simulink model "p4_system_arch_master"  (R2020a)
settings: Solver=VariableStepAuto  StartTime=0.0  StopTime=10.0  RelTol=1e-3
(part 8 of 11)

== system p4_system_arch_master/System 8 : Suspension and Vibration Damping System /motor mount system/support system/Bracket ==

== system p4_system_arch_master/System 8 : Suspension and Vibration Damping System /motor mount system/support system/elastomer ==

== system p4_system_arch_master/System 1 : Electric Motor System /Stator System /1.3 AC HV Connection System  /1.3.1 Connection System /Phase U Connection Ring ==

== system p4_system_arch_master/System 1 : Electric Motor System /Stator System /1.3 AC HV Connection System  /1.3.1 Connection System /Phase V Connection Ring ==

== system p4_system_arch_master/System 1 : Electric Motor System /Stator System /1.3 AC HV Connection System  /1.3.1 Connection System /Phase W Connection Ring ==

== system p4_system_arch_master/System 1 : Electric Motor System /Stator System /1.3 AC HV Connection System  /Isolation System/Isolator Rotor Phase U ==

== system p4_system_arch_master/System 1 : Electric Motor System /Stator System /1.3 AC HV Connection System  /Isolation System/Isolator Rotor Phase U to Phase V ==

== system p4_system_arch_master/System 1 : Electric Motor System /Stator System /1.3 AC HV Connection System  /Isolation System/Isolator Rotor Phase V to Phase W ==

== system p4_system_arch_master/System 10 : Electrical Distribution System /10.1 HV Distribution System /10.1.1	HV DC vehicle interface system/10.1.1.1	HV DC to vehicle connection system/10.1.1.1.1	HV DC Male Connector ==

== system p4_system_arch_master/System 10 : Electrical Distribution System /10.1 HV Distribution System /10.1.1	HV DC vehicle interface system/10.1.1.2	HV DC to inverter connection system/10.1.1.2.1	HV DC Cable Lug "+" ==

== system p4_system_arch_master/System 10 : Electrical Distribution System /10.1 HV Distribution System /10.1.1	HV DC vehicle interface system/10.1.1.2	HV DC to inverter connection system/10.1.1.2.2	HV DC Cable Lug "-"  ==

== system p4_system_arch_master/System 10 : Electrical Distribution System /10.1 HV Distribution System /10.1.1	HV DC vehicle interface system/10.1.1.2	HV DC to inverter connection system/10.1.1.2.3	HV DC Cable Lug "+" Screw ==

== system p4_system_arch_master/System 10 : Electrical Distribution System /10.1 HV Distribution System /10.1.1	HV DC vehicle interface system/10.1.1.2	HV DC to inverter connection system/10.1.1.2.4	HV DC Cable Lug "-" Screw ==

== system p4_system_arch_master/System 10 : Electrical Distribution System /10.1 HV Distribution System /10.1.1	HV DC vehicle interface system/10.1.1.2	HV DC to inverter connection system/10.1.1.2.5	HV DC Cable Lug "+" Washer ==

== system p4_system_arch_master/System 10 : Electrical Distribution System /10.1 HV Distribution System /10.1.1	HV DC vehicle interface system/10.1.1.2	HV DC to inverter connection system/10.1.1.2.6	HV DC Cable Lug "-" Washer ==

== system p4_system_arch_master/System 10 : Electrical Distribution System /10.1 HV Distribution System /10.1.1	HV DC vehicle interface system/10.1.1.3	HV DC Wiring system/10.1.1.3.1	HV DC Wire "+" ==

== system p4_system_arch_master/System 10 : Electrical Distribution System /10.1 HV Distribution System /10.1.1	HV DC vehicle interface system/10.1.1.3	HV DC Wiring system/10.1.1.3.2	HV DC Wire "+" Shielding Braid ==

== system p4_system_arch_master/System 10 : Electrical Distribution System /10.1 HV Distribution System /10.1.1	HV DC vehicle interface system/10.1.1.3	HV DC Wiring system/10.1.1.3.3	HV DC Wire "+" Insulation ==

== system p4_system_arch_master/System 10 : Electrical Distribution System /10.1 HV Distribution System /10.1.1	HV DC vehicle interface system/10.1.1.3	HV DC Wiring system/10.1.1.3.4	HV DC Wire "-" ==

== system p4_system_arch_master/System 10 : Electrical Distribution System /10.1 HV Distribution System /10.1.1	HV DC vehicle interface system/10.1.1.3	HV DC Wiring system/10.1.1.3.5	HV DC Wire "-" Shielding Braid ==

== system p4_system_arch_master/System 10 : Electrical Distribution System /10.1 HV Distribution System /10.1.1	HV DC vehicle interface system/10.1.1.3	HV DC Wiring system/10.1.1.3.6	HV DC Wire "-" Insulation ==

== system p4_system_arch_master/System 10 : Electrical Distribution System /10.1 HV Distribution System /10.1.2	HV AC 3-Phase System (Busbars)/10.1.2.1	HV AC U Busbar System/10.1.2.1.1	HV AC U busbar ==

== system p4_system_arch_master/System 10 : Electrical Distribution System /10.1 HV Distribution System /10.1.2	HV AC 3-Phase System (Busbars)/10.1.2.1	HV AC U Busbar System/10.1.2.1.2	HV AC U busbar to motor bolt ==

== system p4_system_arch_master/System 10 : Electrical Distribution System /10.1 HV Distribution System /10.1.2	HV AC 3-Phase System (Busbars)/10.1.2.1	HV AC U Busbar System/10.1.2.1.3	HV AC U busbar to inverter bolt ==

== system p4_system_arch_master/System 10 : Electrical Distribution System /10.1 HV Distribution System /10.1.2	HV AC 3-Phase System (Busbars)/10.1.2.1	HV AC U Busbar System/10.1.2.1.4	HV AC U busbar to motor washer ==

== system p4_system_arch_master/System 10 : Electrical Distribution System /10.1 HV Distribution System /10.1.2	HV AC 3-Phase System (Busbars)/10.1.2.1	HV AC U Busbar System/10.1.2.1.5	HV AC U busbar to inverter washer ==

== system p4_system_arch_master/System 10 : Electrical Distribution System /10.1 HV Distribution System /10.1.2	HV AC 3-Phase System (Busbars)/10.1.2.1	HV AC U Busbar System/10.1.2.1.6	HV AC U busbar Insulation ==

== system p4_system_arch_master/System 10 : Electrical Distribution System /10.1 HV Distribution System /10.1.2	HV AC 3-Phase System (Busbars)/10.1.2.2	HV AC V Busbar System/10.1.2.2.2	HV AC V busbar to motor bolt ==

== system p4_system_arch_master/System 10 : Electrical Distribution System /10.1 HV Distribution System /10.1.2	HV AC 3-Phase System (Busbars)/10.1.2.2	HV AC V Busbar System/10.1.2.2.3	HV AC V busbar to inverter bolt ==

== system p4_system_arch_master/System 10 : Electrical Distribution System /10.1 HV Distribution System /10.1.2	HV AC 3-Phase System (Busbars)/10.1.2.2	HV AC V Busbar System/10.1.2.2.4	HV AC V busbar to motor washer ==

== system p4_system_arch_master/System 10 : Electrical Distribution System /10.1 HV Distribution System /10.1.2	HV AC 3-Phase System (Busbars)/10.1.2.2	HV AC V Busbar System/10.1.2.2.5	HV AC V busbar to inverter washer ==

== system p4_system_arch_master/System 10 : Electrical Distribution System /10.1 HV Distribution System /10.1.2	HV AC 3-Phase System (Busbars)/10.1.2.2	HV AC V Busbar System/10.1.2.2.6	HV AC V busbar Insulation ==

== system p4_system_arch_master/System 10 : Electrical Distribution System /10.1 HV Distribution System /10.1.2	HV AC 3-Phase System (Busbars)/10.1.2.3	HV AC W Busbar System/10.1.2.3.1	HV AC W busbar ==

== system p4_system_arch_master/System 10 : Electrical Distribution System /10.1 HV Distribution System /10.1.2	HV AC 3-Phase System (Busbars)/10.1.2.3	HV AC W Busbar System/10.1.2.3.2	HV AC W busbar to motor bolt ==

== system p4_system_arch_master/System 10 : Electrical Distribution System /10.1 HV Distribution System /10.1.2	HV AC 3-Phase System (Busbars)/10.1.2.3	HV AC W Busbar System/10.1.2.3.3	HV AC W busbar to inverter bolt ==

== system p4_system_arch_master/System 10 : Electrical Distribution System /10.1 HV Distribution System /10.1.2	HV AC 3-Phase System (Busbars)/10.1.2.3	HV AC W Busbar System/10.1.2.3.4	HV AC W busbar to motor washer ==

== system p4_system_arch_master/System 10 : Electrical Distribution System /10.1 HV Distribution System /10.1.2	HV AC 3-Phase System (Busbars)/10.1.2.3	HV AC W Busbar System/10.1.2.3.5	HV AC W busbar to inverter washer ==

== system p4_system_arch_master/System 10 : Electrical Distribution System /10.1 HV Distribution System /10.1.2	HV AC 3-Phase System (Busbars)/10.1.2.3	HV AC W Busbar System/10.1.2.3.6	HV AC W busbar Insulation ==

== system p4_system_arch_master/System 10 : Electrical Distribution System /10.2 LV Distribution System /10.2.1	Internal LV Loom System/10.2.1.1	Inverter to Motor LV loom system/10.2.1.1.01	Motor LV loom to inverter PCB connector ==

== system p4_system_arch_master/System 10 : Electrical Distribution System /10.2 LV Distribution System /10.2.1	Internal LV Loom System/10.2.1.1	Inverter to Motor LV loom system/PT100 #1 Wire System ==
  "10.2.1.1.18\tPT100 #1 Wire \"Ex+\"" : Subsystem
      settings: PortSchema="{\"entries\":[{\"content\":{\"headerSize\":26,\"margin\":15,\"minimumSpacing\":25,\"sides\":[{\"content\":{\"connectorIds\":[]},\"type\":\"ConnectorPlacement.EquallySpacedRectSide\",\"uuid\":\"f8ee33a9-954f-44c6-a821-b5353f3278fa\"},{\"content\":{\"connectorIds\":[],\"side\":\"RIGHT\"},\"type\":\"ConnectorPlacement.EquallySpacedRectSide\",\"uuid\":\"385f1e4f-1c89-4afc-9c19-76a078cf90bc\"},{\"content\":{\"connectorIds\":[],\"side\":\"TOP\"},\"type\":\"ConnectorPlacement.EquallySpacedRectSide\",\"uuid\":\"fc91fa49-46f5-4ba7-960e-7bda5e0416d1\"}]},\"type\":\"ConnectorPlacement.EquallySpacedConnector\",\"uuid\":\"4bf08bc6-c7ce-47fb-af04-cd9d2b5f8092\"}],\"packageUris\":[\"http://schema.mathworks.com/mf0/Connector/19700101\"],\"version\":\"1.0\"}"
  "10.2.1.1.19\tPT100 #1 Wire \"Ex-\"" : Subsystem
      settings: PortSchema="{\"entries\":[{\"content\":{\"headerSize\":26,\"margin\":15,\"minimumSpacing\":25,\"sides\":[{\"content\":{\"connectorIds\":[]},\"type\":\"ConnectorPlacement.EquallySpacedRectSide\",\"uuid\":\"f8ee33a9-954f-44c6-a821-b5353f3278fa\"},{\"content\":{\"connectorIds\":[],\"side\":\"RIGHT\"},\"type\":\"ConnectorPlacement.EquallySpacedRectSide\",\"uuid\":\"385f1e4f-1c89-4afc-9c19-76a078cf90bc\"},{\"content\":{\"connectorIds\":[],\"side\":\"TOP\"},\"type\":\"ConnectorPlacement.EquallySpacedRectSide\",\"uuid\":\"fc91fa49-46f5-4ba7-960e-7bda5e0416d1\"}]},\"type\":\"ConnectorPlacement.EquallySpacedConnector\",\"uuid\":\"4bf08bc6-c7ce-47fb-af04-cd9d2b5f8092\"}],\"packageUris\":[\"http://schema.mathworks.com/mf0/Connector/19700101\"],\"version\":\"1.0\"}"
  "10.2.1.1.20\tPT100 #1 Wire \"Ex+\" Insulation" : Subsystem
      settings: PortSchema="{\"entries\":[{\"content\":{\"headerSize\":26,\"margin\":15,\"minimumSpacing\":25,\"sides\":[{\"content\":{\"connectorIds\":[]},\"type\":\"ConnectorPlacement.EquallySpacedRectSide\",\"uuid\":\"f8ee33a9-954f-44c6-a821-b5353f3278fa\"},{\"content\":{\"connectorIds\":[],\"side\":\"RIGHT\"},\"type\":\"ConnectorPlacement.EquallySpacedRectSide\",\"uuid\":\"385f1e4f-1c89-4afc-9c19-76a078cf90bc\"},{\"content\":{\"connectorIds\":[],\"side\":\"TOP\"},\"type\":\"ConnectorPlacement.EquallySpacedRectSide\",\"uuid\":\"fc91fa49-46f5-4ba7-960e-7bda5e0416d1\"}]},\"type\":\"ConnectorPlacement.EquallySpacedConnector\",\"uuid\":\"4bf08bc6-c7ce-47fb-af04-cd9d2b5f8092\"}],\"packageUris\":[\"http://schema.mathworks.com/mf0/Connector/19700101\"],\"version\":\"1.0\"}"
  "10.2.1.1.21\tPT100 #1 Wire \"Ex-\" Insulation" : Subsystem
      settings: PortSchema="{\"entries\":[{\"content\":{\"headerSize\":26,\"margin\":15,\"minimumSpacing\":25,\"sides\":[{\"content\":{\"connectorIds\":[]},\"type\":\"ConnectorPlacement.EquallySpacedRectSide\",\"uuid\":\"f8ee33a9-954f-44c6-a821-b5353f3278fa\"},{\"content\":{\"connectorIds\":[],\"side\":\"RIGHT\"},\"type\":\"ConnectorPlacement.EquallySpacedRectSide\",\"uuid\":\"385f1e4f-1c89-4afc-9c19-76a078cf90bc\"},{\"content\":{\"connectorIds\":[],\"side\":\"TOP\"},\"type\":\"ConnectorPlacement.EquallySpacedRectSide\",\"uuid\":\"fc91fa49-46f5-4ba7-960e-7bda5e0416d1\"}]},\"type\":\"ConnectorPlacement.EquallySpacedConnector\",\"uuid\":\"4bf08bc6-c7ce-47fb-af04-cd9d2b5f8092\"}],\"packageUris\":[\"http://schema.mathworks.com/mf0/Connector/19700101\"],\"version\":\"1.0\"}"
  "10.2.1.1.22\tPT100 #1 Wire pair \"Ex\" shielding braid" : Subsystem
      settings: PortSchema="{\"entries\":[{\"content\":{\"headerSize\":26,\"margin\":15,\"minimumSpacing\":25,\"sides\":[{\"content\":{\"connectorIds\":[]},\"type\":\"ConnectorPlacement.EquallySpacedRectSide\",\"uuid\":\"f8ee33a9-954f-44c6-a821-b5353f3278fa\"},{\"content\":{\"connectorIds\":[],\"side\":\"RIGHT\"},\"type\":\"ConnectorPlacement.EquallySpacedRectSide\",\"uuid\":\"385f1e4f-1c89-4afc-9c19-76a078cf90bc\"},{\"content\":{\"connectorIds\":[],\"side\":\"TOP\"},\"type\":\"ConnectorPlacement.EquallySpacedRectSide\",\"uuid\":\"fc91fa49-46f5-4ba7-960e-7bda5e0416d1\"}]},\"type\":\"ConnectorPlacement.EquallySpacedConnector\",\"uuid\":\"4bf08bc6-c7ce-47fb-af04-cd9d2b5f8092\"}],\"packageUris\":[\"http://schema.mathworks.com/mf0/Connector/19700101\"],\"version\":\"1.0\"}"

== system p4_system_arch_master/System 10 : Electrical Distribution System /10.2 LV Distribution System /10.2.1	Internal LV Loom System/10.2.1.1	Inverter to Motor LV loom system/PT100 #2 Wire System ==
  "10.2.1.1.23\tPT100 #2 Wire \"Ex+\"" : Subsystem
      settings: PortSchema="{\"entries\":[{\"content\":{\"headerSize\":26,\"margin\":15,\"minimumSpacing\":25,\"sides\":[{\"content\":{\"connectorIds\":[]},\"type\":\"ConnectorPlacement.EquallySpacedRectSide\",\"uuid\":\"f8ee33a9-954f-44c6-a821-b5353f3278fa\"},{\"content\":{\"connectorIds\":[],\"side\":\"RIGHT\"},\"type\":\"ConnectorPlacement.EquallySpacedRectSide\",\"uuid\":\"385f1e4f-1c89-4afc-9c19-76a078cf90bc\"},{\"content\":{\"connectorIds\":[],\"side\":\"TOP\"},\"type\":\"ConnectorPlacement.EquallySpacedRectSide\",\"uuid\":\"fc91fa49-46f5-4ba7-960e-7bda5e0416d1\"}]},\"type\":\"ConnectorPlacement.EquallySpacedConnector\",\"uuid\":\"4bf08bc6-c7ce-47fb-af04-cd9d2b5f8092\"}],\"packageUris\":[\"http://schema.mathworks.com/mf0/Connector/19700101\"],\"version\":\"1.0\"}"
  "10.2.1.1.24\tPT100 #2 Wire \"Ex-\"" : Subsystem
      settings: PortSchema="{\"entries\":[{\"content\":{\"headerSize\":26,\"margin\":15,\"minimumSpacing\":25,\"sides\":[{\"content\":{\"connectorIds\":[]},\"type\":\"ConnectorPlacement.EquallySpacedRectSide\",\"uuid\":\"f8ee33a9-954f-44c6-a821-b5353f3278fa\"},{\"content\":{\"connectorIds\":[],\"side\":\"RIGHT\"},\"type\":\"ConnectorPlacement.EquallySpacedRectSide\",\"uuid\":\"385f1e4f-1c89-4afc-9c19-76a078cf90bc\"},{\"content\":{\"connectorIds\":[],\"side\":\"TOP\"},\"type\":\"ConnectorPlacement.EquallySpacedRectSide\",\"uuid\":\"fc91fa49-46f5-4ba7-960e-7bda5e0416d1\"}]},\"type\":\"ConnectorPlacement.EquallySpacedConnector\",\"uuid\":\"4bf08bc6-c7ce-47fb-af04-cd9d2b5f8092\"}],\"packageUris\":[\"http://schema.mathworks.com/mf0/Connector/19700101\"],\"version\":\"1.0\"}"
  "10.2.1.1.25\tPT100 #2 Wire \"Ex+\" Insulation" : Subsystem
      settings: PortSchema="{\"entries\":[{\"content\":{\"headerSize\":26,\"margin\":15,\"minimumSpacing\":25,\"sides\":[{\"content\":{\"connectorIds\":[]},\"type\":\"ConnectorPlacement.EquallySpacedRectSide\",\"uuid\":\"f8ee33a9-954f-44c6-a821-b5353f3278fa\"},{\"content\":{\"connectorIds\":[],\"side\":\"RIGHT\"},\"type\":\"ConnectorPlacement.EquallySpacedRectSide\",\"uuid\":\"385f1e4f-1c89-4afc-9c19-76a078cf90bc\"},{\"content\":{\"connectorIds\":[],\"side\":\"TOP\"},\"type\":\"ConnectorPlacement.EquallySpacedRectSide\",\"uuid\":\"fc91fa49-46f5-4ba7-960e-7bda5e0416d1\"}]},\"type\":\"ConnectorPlacement.EquallySpacedConnector\",\"uuid\":\"4bf08bc6-c7ce-47fb-af04-cd9d2b5f8092\"}],\"packageUris\":[\"http://schema.mathworks.com/mf0/Connector/19700101\"],\"version\":\"1.0\"}"
  "10.2.1.1.26\tPT100 #2 Wire \"Ex-\" Insulation" : Subsystem
      settings: PortSchema="{\"entries\":[{\"content\":{\"headerSize\":26,\"margin\":15,\"minimumSpacing\":25,\"sides\":[{\"content\":{\"connectorIds\":[]},\"type\":\"ConnectorPlacement.EquallySpacedRectSide\",\"uuid\":\"f8ee33a9-954f-44c6-a821-b5353f3278fa\"},{\"content\":{\"connectorIds\":[],\"side\":\"RIGHT\"},\"type\":\"ConnectorPlacement.EquallySpacedRectSide\",\"uuid\":\"385f1e4f-1c89-4afc-9c19-76a078cf90bc\"},{\"content\":{\"connectorIds\":[],\"side\":\"TOP\"},\"type\":\"ConnectorPlacement.EquallySpacedRectSide\",\"uuid\":\"fc91fa49-46f5-4ba7-960e-7bda5e0416d1\"}]},\"type\":\"ConnectorPlacement.EquallySpacedConnector\",\"uuid\":\"4bf08bc6-c7ce-47fb-af04-cd9d2b5f8092\"}],\"packageUris\":[\"http://schema.mathworks.com/mf0/Connector/19700101\"],\"version\":\"1.0\"}"
  "10.2.1.1.27\tPT100 #2 Wire pair \"Ex\" shielding braid" : Subsystem
      settings: PortSchema="{\"entries\":[{\"content\":{\"headerSize\":26,\"margin\":15,\"minimumSpacing\":25,\"sides\":[{\"content\":{\"connectorIds\":[]},\"type\":\"ConnectorPlacement.EquallySpacedRectSide\",\"uuid\":\"f8ee33a9-954f-44c6-a821-b5353f3278fa\"},{\"content\":{\"connectorIds\":[],\"side\":\"RIGHT\"},\"type\":\"ConnectorPlacement.EquallySpacedRectSide\",\"uuid\":\"385f1e4f-1c89-4afc-9c19-76a078cf90bc\"},{\"content\":{\"connectorIds\":[],\"side\":\"TOP\"},\"type\":\"ConnectorPlacement.EquallySpacedRectSide\",\"uuid\":\"fc91fa49-46f5-4ba7-960e-7bda5e0416d1\"}]},\"type\":\"ConnectorPlacement.EquallySpacedConnector\",\"uuid\":\"4bf08bc6-c7ce-47fb-af04-cd9d2b5f8092\"}],\"packageUris\":[\"http://schema.mathworks.com/mf0/Connector/19700101\"],\"version\":\"1.0\"}"

== system p4_system_arch_master/System 10 : Electrical Distribution System /10.2 LV Distribution System /10.2.1	Internal LV Loom System/10.2.1.1	Inverter to Motor LV loom system/Resolver sensor System ==
  10.2.1.1.02	Resolver sensor connector : Subsystem
      settings: PortSchema="{\"entries\":[{\"content\":{\"headerSize\":26,\"margin\":15,\"minimumSpacing\":25,\"sides\":[{\"content\":{\"connectorIds\":[]},\"type\":\"ConnectorPlacement.EquallySpacedRectSide\",\"uuid\":\"f8ee33a9-954f-44c6-a821-b5353f3278fa\"},{\"content\":{\"connectorIds\":[],\"side\":\"RIGHT\"},\"type\":\"ConnectorPlacement.EquallySpacedRectSide\",\"uuid\":\"385f1e4f-1c89-4afc-9c19-76a078cf90bc\"},{\"content\":{\"connectorIds\":[],\"side\":\"TOP\"},\"type\":\"ConnectorPlacement.EquallySpacedRectSide\",\"uuid\":\"fc91fa49-46f5-4ba7-960e-7bda5e0416d1\"}]},\"type\":\"ConnectorPlacement.EquallySpacedConnector\",\"uuid\":\"4bf08bc6-c7ce-47fb-af04-cd9d2b5f8092\"}],\"packageUris\":[\"http://schema.mathworks.com/mf0/Connector/19700101\"],\"version\":\"1.0\"}"
  10.2.1.1.03	Resolver sensor  Wires : Subsystem
      settings: PortSchema="{\"entries\":[{\"content\":{\"headerSize\":26,\"margin\":15,\"minimumSpacing\":25,\"sides\":[{\"content\":{\"connectorIds\":[]},\"type\":\"ConnectorPlacement.EquallySpacedRectSide\",\"uuid\":\"f8ee33a9-954f-44c6-a821-b5353f3278fa\"},{\"content\":{\"connectorIds\":[],\"side\":\"RIGHT\"},\"type\":\"ConnectorPlacement.EquallySpacedRectSide\",\"uuid\":\"385f1e4f-1c89-4afc-9c19-76a078cf90bc\"},{\"content\":{\"connectorIds\":[],\"side\":\"TOP\"},\"type\":\"ConnectorPlacement.EquallySpacedRectSide\",\"uuid\":\"fc91fa49-46f5-4ba7-960e-7bda5e0416d1\"}]},\"type\":\"ConnectorPlacement.EquallySpacedConnector\",\"uuid\":\"4bf08bc6-c7ce-47fb-af04-cd9d2b5f8092\"}],\"packageUris\":[\"http://schema.mathworks.com/mf0/Connector/19700101\"],\"version\":\"1.0\"}"

== system p4_system_arch_master/System 10 : Electrical Distribution System /10.2 LV Distribution System /10.2.1	Internal LV Loom System/10.2.1.2	Inverter to Inverter LV connector loom system/10.2.1.2.01	Inverter LV external connector ==

== system p4_system_arch_master/System 10 : Electrical Distribution System /10.2 LV Distribution System /10.2.1	Internal LV Loom System/10.2.1.2	Inverter to Inverter LV connector loom system/10.2.1.2.02	Inverter internal loom to PCB connector ==

== system p4_system_arch_master/System 10 : Electrical Distribution System /10.2 LV Distribution System /10.2.1	Internal LV Loom System/10.2.1.2	Inverter to Inverter LV connector loom system/Inverter Internal Wires ==
  CAN1_H Wire : Subsystem
      settings: PortSchema="{\"entries\":[{\"content\":{\"headerSize\":26,\"margin\":15,\"minimumSpacing\":25,\"sides\":[{\"content\":{\"connectorIds\":[]},\"type\":\"ConnectorPlacement.EquallySpacedRectSide\",\"uuid\":\"f8ee33a9-954f-44c6-a821-b5353f3278fa\"},{\"content\":{\"connectorIds\":[],\"side\":\"RIGHT\"},\"type\":\"ConnectorPlacement.EquallySpacedRectSide\",\"uuid\":\"385f1e4f-1c89-4afc-9c19-76a078cf90bc\"},{\"content\":{\"connectorIds\":[],\"side\":\"TOP\"},\"type\":\"ConnectorPlacement.EquallySpacedRectSide\",\"uuid\":\"fc91fa49-46f5-4ba7-960e-7bda5e0416d1\"}]},\"type\":\"ConnectorPlacement.EquallySpacedConnector\",\"uuid\":\"4bf08bc6-c7ce-47fb-af04-cd9d2b5f8092\"}],\"packageUris\":[\"http://schema.mathworks.com/mf0/Connector/19700101\"],\"version\":\"1.0\"}"
  CAN1_L Wire : Subsystem
      settings: PortSchema="{\"entries\":[{\"content\":{\"headerSize\":26,\"margin\":15,\"minimumSpacing\":25,\"sides\":[{\"content\":{\"connectorIds\":[]},\"type\":\"ConnectorPlacement.EquallySpacedRectSide\",\"uuid\":\"f8ee33a9-954f-44c6-a821-b5353f3278fa\"},{\"content\":{\"connectorIds\":[],\"side\":\"RIGHT\"},\"type\":\"ConnectorPlacement.EquallySpacedRectSide\",\"uuid\":\"385f1e4f-1c89-4afc-9c19-76a078cf90bc\"},{\"content\":{\"connectorIds\":[],\"side\":\"TOP\"},\"type\":\"ConnectorPlacement.EquallySpacedRectSide\",\"uuid\":\"fc91fa49-46f5-4ba7-960e-7bda5e0416d1\"}]},\"type\":\"ConnectorPlacement.EquallySpacedConnector\",\"uuid\":\"4bf08bc6-c7ce-47fb-af04-cd9d2b5f8092\"}],\"packageUris\":[\"http://schema.mathworks.com/mf0/Connector/19700101\"],\"version\":\"1.0\"}"
  CAN2_H Wire : Subsystem
      settings: PortSchema="{\"entries\":[{\"content\":{\"headerSize\":26,\"margin\":15,\"minimumSpacing\":25,\"sides\":[{\"content\":{\"connectorIds\":[]},\"type\":\"ConnectorPlacement.EquallySpacedRectSide\",\"uuid\":\"f8ee33a9-954f-44c6-a821-b5353f3278fa\"},{\"content\":{\"connectorIds\":[],\"side\":\"RIGHT\"},\"type\":\"ConnectorPlacement.EquallySpacedRectSide\",\"uuid\":\"385f1e4f-1c89-4afc-9c19-76a078cf90bc\"},{\"content\":{\"connectorIds\":[],\"side\":\"TOP\"},\"type\":\"ConnectorPlacement.EquallySpacedRectSide\",\"uuid\":\"fc91fa49-46f5-4ba7-960e-7bda5e0416d1\"}]},\"type\":\"ConnectorPlacement.EquallySpacedConnector\",\"uuid\":\"4bf08bc6-c7ce-47fb-af04-cd9d2b5f8092\"}],\"packageUris\":[\"http://schema.mathworks.com/mf0/Connector/19700101\"],\"version\":\"1.0\"}"
  "CAN2_L Wire " : Subsystem
      settings: PortSchema="{\"entries\":[{\"content\":{\"headerSize\":26,\"margin\":15,\"minimumSpacing\":25,\"sides\":[{\"content\":{\"connectorIds\":[]},\"type\":\"ConnectorPlacement.EquallySpacedRectSide\",\"uuid\":\"f8ee33a9-954f-44c6-a821-b5353f3278fa\"},{\"content\":{\"connectorIds\":[],\"side\":\"RIGHT\"},\"type\":\"ConnectorPlacement.EquallySpacedRectSide\",\"uuid\":\"385f1e4f-1c89-4afc-9c19-76a078cf90bc\"},{\"content\":{\"connectorIds\":[],\"side\":\"TOP\"},\"type\":\"ConnectorPlacement.EquallySpacedRectSide\",\"uuid\":\"fc91fa49-46f5-4ba7-960e-7bda5e0416d1\"}]},\"type\":\"ConnectorPlacement.EquallySpacedConnector\",\"uuid\":\"4bf08bc6-c7ce-47fb-af04-cd9d2b5f8092\"}],\"packageUris\":[\"http://schema.mathworks.com/mf0/Connector/19700101\"],\"version\":\"1.0\"}"
  DIN1 Wire : Subsystem
      settings: PortSchema="{\"entries\":[{\"content\":{\"headerSize\":26,\"margin\":15,\"minimumSpacing\":25,\"sides\":[{\"content\":{\"connectorIds\":[]},\"type\":\"ConnectorPlacement.EquallySpacedRectSide\",\"uuid\":\"f8ee33a9-954f-44c6-a821-b5353f3278fa\"},{\"content\":{\"connectorIds\":[],\"side\":\"RIGHT\"},\"type\":\"ConnectorPlacement.EquallySpacedRectSide\",\"uuid\":\"385f1e4f-1c89-4afc-9c19-76a078cf90bc\"},{\"content\":{\"connectorIds\":[],\"side\":\"TOP\"},\"type\":\"ConnectorPlacement.EquallySpacedRectSide\",\"uuid\":\"fc91fa49-46f5-4ba7-960e-7bda5e0416d1\"}]},\"type\":\"ConnectorPlacement.EquallySpacedConnector\",\"uuid\":\"4bf08bc6-c7ce-47fb-af04-cd9d2b5f8092\"}],\"packageUris\":[\"http://schema.mathworks.com/mf0/Connector/19700101\"],\"version\":\"1.0\"}"
  DIN2 Wire : Subsystem
      settings: PortSchema="{\"entries\":[{\"content\":{\"headerSize\":26,\"margin\":15,\"minimumSpacing\":25,\"sides\":[{\"content\":{\"connectorIds\":[]},\"type\":\"ConnectorPlacement.EquallySpacedRectSide\",\"uuid\":\"f8ee33a9-954f-44c6-a821-b5353f3278fa\"},{\"content\":{\"connectorIds\":[],\"side\":\"RIGHT\"},\"type\":\"ConnectorPlacement.EquallySpacedRectSide\",\"uuid\":\"385f1e4f-1c89-4afc-9c19-76a078cf90bc\"},{\"content\":{\"connectorIds\":[],\"side\":\"TOP\"},\"type\":\"ConnectorPlacement.EquallySpacedRectSide\",\"uuid\":\"fc91fa49-46f5-4ba7-960e-7bda5e0416d1\"}]},\"type\":\"ConnectorPlacement.EquallySpacedConnector\",\"uuid\":\"4bf08bc6-c7ce-47fb-af04-cd9d2b5f8092\"}],\"packageUris\":[\"http://schema.mathworks.com/mf0/Connector/19700101\"],\"version\":\"1.0\"}"
  DOUT1 Wire : Subsystem
      settings: PortSchema="{\"entries\":[{\"content\":{\"headerSize\":26,\"margin\":15,\"minimumSpacing\":25,\"sides\":[{\"content\":{\"connectorIds\":[]},\"type\":\"ConnectorPlacement.EquallySpacedRectSide\",\"uuid\":\"f8ee33a9-954f-44c6-a821-b5353f3278fa\"},{\"content\":{\"connectorIds\":[],\"side\":\"RIGHT\"},\"type\":\"ConnectorPlacement.EquallySpacedRectSide\",\"uuid\":\"385f1e4f-1c89-4afc-9c19-76a078cf90bc\"},{\"content\":{\"connectorIds\":[],\"side\":\"TOP\"},\"type\":\"ConnectorPlacement.EquallySpacedRectSide\",\"uuid\":\"fc91fa49-46f5-4ba7-960e-7bda5e0416d1\"}]},\"type\":\"ConnectorPlacement.EquallySpacedConnector\",\"uuid\":\"4bf08bc6-c7ce-47fb-af04-cd9d2b5f8092\"}],\"packageUris\":[\"http://schema.mathworks.com/mf0/Connector/19700101\"],\"version\":\"1.0\"}"
  DOUT2 Wire : Subsystem
      settings: PortSchema="{\"entries\":[{\"content\":{\"headerSize\":26,\"margin\":15,\"minimumSpacing\":25,\"sides\":[{\"content\":{\"connectorIds\":[]},\"type\":\"ConnectorPlacement.EquallySpacedRectSide\",\"uuid\":\"f8ee33a9-954f-44c6-a821-b5353f3278fa\"},{\"content\":{\"connectorIds\":[],\"side\":\"RIGHT\"},\"type\":\"ConnectorPlacement.EquallySpacedRectSide\",\"uuid\":\"385f1e4f-1c89-4afc-9c19-76a078cf90bc\"},{\"content\":{\"connectorIds\":[],\"side\":\"TOP\"},\"type\":\"ConnectorPlacement.EquallySpacedRectSide\",\"uuid\":\"fc91fa49-46f5-4ba7-960e-7bda5e0416d1\"}]},\"type\":\"ConnectorPlacement.EquallySpacedConnector\",\"uuid\":\"4bf08bc6-c7ce-47fb-af04-cd9d2b5f8092\"}],\"packageUris\":[\"http://schema.mathworks.com/mf0/Connector/19700101\"],\"version\":\"1.0\"}"
  ETH_N Wire : Subsystem
      settings: PortSchema="{\"entries\":[{\"content\":{\"headerSize\":26,\"margin\":15,\"minimumSpacing\":25,\"sides\":[{\"content\":{\"connectorIds\":[]},\"type\":\"ConnectorPlacement.EquallySpacedRectSide\",\"uuid\":\"f8ee33a9-954f-44c6-a821-b5353f3278fa\"},{\"content\":{\"connectorIds\":[],\"side\":\"RIGHT\"},\"type\":\"ConnectorPlacement.EquallySpacedRectSide\",\"uuid\":\"385f1e4f-1c89-4afc-9c19-76a078cf90bc\"},{\"content\":{\"connectorIds\":[],\"side\":\"TOP\"},\"type\":\"ConnectorPlacement.EquallySpacedRectSide\",\"uuid\":\"fc91fa49-46f5-4ba7-960e-7bda5e0416d1\"}]},\"type\":\"ConnectorPlacement.EquallySpacedConnector\",\"uuid\":\"4bf08bc6-c7ce-47fb-af04-cd9d2b5f8092\"}],\"packageUris\":[\"http://schema.mathworks.com/mf0/Connector/19700101\"],\"version\":\"1.0\"}"
  ETH_P Wire : Subsystem
      settings: PortSchema="{\"entries\":[{\"content\":{\"headerSize\":26,\"margin\":15,\"minimumSpacing\":25,\"sides\":[{\"content\":{\"connectorIds\":[]},\"type\":\"ConnectorPlacement.EquallySpacedRectSide\",\"uuid\":\"f8ee33a9-954f-44c6-a821-b5353f3278fa\"},{\"content\":{\"connectorIds\":[],\"side\":\"RIGHT\"},\"type\":\"ConnectorPlacement.EquallySpacedRectSide\",\"uuid\":\"385f1e4f-1c89-4afc-9c19-76a078cf90bc\"},{\"content\":{\"connectorIds\":[],\"side\":\"TOP\"},\"type\":\"ConnectorPlacement.EquallySpacedRectSide\",\"uuid\":\"fc91fa49-46f5-4ba7-960e-7bda5e0416d1\"}]},\"type\":\"ConnectorPlacement.EquallySpacedConnector\",\"uuid\":\"4bf08bc6-c7ce-47fb-af04-cd9d2b5f8092\"}],\"packageUris\":[\"http://schema.mathworks.com/mf0/Connector/19700101\"],\"version\":\"1.0\"}"
  "GND Wire " : Subsystem
      settings: PortSchema="{\"entries\":[{\"content\":{\"headerSize\":26,\"margin\":15,\"minimumSpacing\":25,\"sides\":[{\"content\":{\"connectorIds\":[]},\"type\":\"ConnectorPlacement.EquallySpacedRectSide\",\"uuid\":\"f8ee33a9-954f-44c6-a821-b5353f3278fa\"},{\"content\":{\"connectorIds\":[],\"side\":\"RIGHT\"},\"type\":\"ConnectorPlacement.EquallySpacedRectSide\",\"uuid\":\"385f1e4f-1c89-4afc-9c19-76a078cf90bc\"},{\"content\":{\"connectorIds\":[],\"side\":\"TOP\"},\"type\":\"ConnectorPlacement.EquallySpacedRectSide\",\"uuid\":\"fc91fa49-46f5-4ba7-960e-7bda5e0416d1\"}]},\"type\":\"ConnectorPlacement.EquallySpacedConnector\",\"uuid\":\"4bf08bc6-c7ce-47fb-af04-cd9d2b5f8092\"}],\"packageUris\":[\"http://schema.mathworks.com/mf0/Connector/19700101\"],\"version\":\"1.0\"}"
  VCC Wire : Subsystem
      settings: PortSchema="{\"entries\":[{\"content\":{\"headerSize\":26,\"margin\":15,\"minimumSpacing\":25,\"sides\":[{\"content\":{\"connectorIds\":[]},\"type\":\"ConnectorPlacement.EquallySpacedRectSide\",\"uuid\":\"f8ee33a9-954f-44c6-a821-b5353f3278fa\"},{\"content\":{\"connectorIds\":[],\"side\":\"RIGHT\"},\"type\":\"ConnectorPlacement.EquallySpacedRectSide\",\"uuid\":\"385f1e4f-1c89-4afc-9c19-76a078cf90bc\"},{\"content\":{\"connectorIds\":[],\"side\":\"TOP\"},\"type\":\"ConnectorPlacement.EquallySpacedRectSide\",\"uuid\":\"fc91fa49-46f5-4ba7-960e-7bda5e0416d1\"}]},\"type\":\"ConnectorPlacement.EquallySpacedConnector\",\"uuid\":\"4bf08bc6-c7ce-47fb-af04-cd9d2b5f8092\"}],\"packageUris\":[\"http://schema.mathworks.com/mf0/Connector/19700101\"],\"version\":\"1.0\"}"

== system p4_system_arch_master/System 10 : Electrical Distribution System /10.2 LV Distribution System /10.2.1	Internal LV Loom System/10.2.1.3	Internal LV loom restraining system/10.2.1.3.1	Cable clips ==

== system p4_system_arch_master/System 10 : Electrical Distribution System /10.2 LV Distribution System /10.2.2	External LV Loom System/10.2.2.1	External LV loom connectors system/10.2.2.1.01	Main LV connector IDU to vehicle  ==

== system p4_system_arch_master/System 10 : Electrical Distribution System /10.2 LV Distribution System /10.2.2	External LV Loom System/10.2.2.1	External LV loom connectors system/10.2.2.1.02	Inverter cable connector ==

== system p4_system_arch_master/System 10 : Electrical Distribution System /10.2 LV Distribution System /10.2.2	External LV Loom System/10.2.2.1	External LV loom connectors system/10.2.2.1.03	I//O module X1 cable connector ==

== system p4_system_arch_master/System 10 : Electrical Distribution System /10.2 LV Distribution System /10.2.2	External LV Loom System/10.2.2.1	External LV loom connectors system/10.2.2.1.04	I//O module X2 cable connector ==

== system p4_system_arch_master/System 10 : Electrical Distribution System /10.2 LV Distribution System /10.2.2	External LV Loom System/10.2.2.1	External LV loom connectors system/10.2.2.1.05	Oil temperature sensor connector ==

== system p4_system_arch_master/System 10 : Electrical Distribution System /10.2 LV Distribution System /10.2.2	External LV Loom System/10.2.2.1	External LV loom connectors system/10.2.2.1.06	Input speed sensor connector ==

== system p4_system_arch_master/System 10 : Electrical Distribution System /10.2 LV Distribution System /10.2.2	External LV Loom System/10.2.2.1	External LV loom connectors system/10.2.2.1.07	Output speed sensor connector ==

== system p4_system_arch_master/System 10 : Electrical Distribution System /10.2 LV Distribution System /10.2.2	External LV Loom System/10.2.2.1	External LV loom connectors system/10.2.2.1.08	Shifting actuator Cable terminal "+" ==

== system p4_system_arch_master/System 10 : Electrical Distribution System /10.2 LV Distribution System /10.2.2	External LV Loom System/10.2.2.1	External LV loom connectors system/10.2.2.1.09	Shifting actuator Cable terminal "-" ==

== system p4_system_arch_master/System 10 : Electrical Distribution System /10.2 LV Distribution System /10.2.2	External LV Loom System/10.2.2.2	External LV loom wiring system/Barrel Cam Position Speed Sensor Wires  ==
  "10.2.2.2.52\tBarrel cam position sensor wire \"5V Ref\"" : Subsystem
      settings: PortSchema="{\"entries\":[{\"content\":{\"headerSize\":26,\"margin\":15,\"minimumSpacing\":25,\"sides\":[{\"content\":{\"connectorIds\":[]},\"type\":\"ConnectorPlacement.EquallySpacedRectSide\",\"uuid\":\"f8ee33a9-954f-44c6-a821-b5353f3278fa\"},{\"content\":{\"connectorIds\":[],\"side\":\"RIGHT\"},\"type\":\"ConnectorPlacement.EquallySpacedRectSide\",\"uuid\":\"385f1e4f-1c89-4afc-9c19-76a078cf90bc\"},{\"content\":{\"connectorIds\":[],\"side\":\"TOP\"},\"type\":\"ConnectorPlacement.EquallySpacedRectSide\",\"uuid\":\"fc91fa49-46f5-4ba7-960e-7bda5e0416d1\"}]},\"type\":\"ConnectorPlacement.EquallySpacedConnector\",\"uuid\":\"4bf08bc6-c7ce-47fb-af04-cd9d2b5f8092\"}],\"packageUris\":[\"http://schema.mathworks.com/mf0/Connector/19700101\"],\"version\":\"1.0\"}"
  "10.2.2.2.53\tBarrel cam position sensor wire \"GND\"" : Subsystem
      settings: PortSchema="{\"entries\":[{\"content\":{\"headerSize\":26,\"margin\":15,\"minimumSpacing\":25,\"sides\":[{\"content\":{\"connectorIds\":[]},\"type\":\"ConnectorPlacement.EquallySpacedRectSide\",\"uuid\":\"f8ee33a9-954f-44c6-a821-b5353f3278fa\"},{\"content\":{\"connectorIds\":[],\"side\":\"RIGHT\"},\"type\":\"ConnectorPlacement.EquallySpacedRectSide\",\"uuid\":\"385f1e4f-1c89-4afc-9c19-76a078cf90bc\"},{\"content\":{\"connectorIds\":[],\"side\":\"TOP\"},\"type\":\"ConnectorPlacement.EquallySpacedRectSide\",\"uuid\":\"fc91fa49-46f5-4ba7-960e-7bda5e0416d1\"}]},\"type\":\"ConnectorPlacement.EquallySpacedConnector\",\"uuid\":\"4bf08bc6-c7ce-47fb-af04-cd9d2b5f8092\"}],\"packageUris\":[\"http://schema.mathworks.com/mf0/Connector/19700101\"],\"version\":\"1.0\"}"
  "10.2.2.2.54\tBarrel cam position sensor wire \"Analog Output 1\"" : Subsystem
      settings: PortSchema="{\"entries\":[{\"content\":{\"headerSize\":26,\"margin\":15,\"minimumSpacing\":25,\"sides\":[{\"content\":{\"connectorIds\":[]},\"type\":\"ConnectorPlacement.EquallySpacedRectSide\",\"uuid\":\"f8ee33a9-954f-44c6-a821-b5353f3278fa\"},{\"content\":{\"connectorIds\":[],\"side\":\"RIGHT\"},\"type\":\"ConnectorPlacement.EquallySpacedRectSide\",\"uuid\":\"385f1e4f-1c89-4afc-9c19-76a078cf90bc\"},{\"content\":{\"connectorIds\":[],\"side\":\"TOP\"},\"type\":\"ConnectorPlacement.EquallySpacedRectSide\",\"uuid\":\"fc91fa49-46f5-4ba7-960e-7bda5e0416d1\"}]},\"type\":\"ConnectorPlacement.EquallySpacedConnector\",\"uuid\":\"4bf08bc6-c7ce-47fb-af04-cd9d2b5f8092\"}],\"packageUris\":[\"http://schema.mathworks.com/mf0/Connector/19700101\"],\"version\":\"1.0\"}"
  "10.2.2.2.55\tBarrel cam position sensor wire \"Analog Output 2\"" : Subsystem
      settings: PortSchema="{\"entries\":[{\"content\":{\"headerSize\":26,\"margin\":15,\"minimumSpacing\":25,\"sides\":[{\"content\":{\"connectorIds\":[]},\"type\":\"ConnectorPlacement.EquallySpacedRectSide\",\"uuid\":\"f8ee33a9-954f-44c6-a821-b5353f3278fa\"},{\"content\":{\"connectorIds\":[],\"side\":\"RIGHT\"},\"type\":\"ConnectorPlacement.EquallySpacedRectSide\",\"uuid\":\"385f1e4f-1c89-4afc-9c19-76a078cf90bc\"},{\"content\":{\"connectorIds\":[],\"side\":\"TOP\"},\"type\":\"ConnectorPlacement.EquallySpacedRectSide\",\"uuid\":\"fc91fa49-46f5-4ba7-960e-7bda5e0416d1\"}]},\"type\":\"ConnectorPlacement.EquallySpacedConnector\",\"uuid\":\"4bf08bc6-c7ce-47fb-af04-cd9d2b5f8092\"}],\"packageUris\":[\"http://schema.mathworks.com/mf0/Connector/19700101\"],\"version\":\"1.0\"}"
  "10.2.2.2.56\tBarrel cam position sensor wire \"5V Ref\" insulation" : Subsystem
      settings: PortSchema="{\"entries\":[{\"content\":{\"headerSize\":26,\"margin\":15,\"minimumSpacing\":25,\"sides\":[{\"content\":{\"connectorIds\":[]},\"type\":\"ConnectorPlacement.EquallySpacedRectSide\",\"uuid\":\"f8ee33a9-954f-44c6-a821-b5353f3278fa\"},{\"content\":{\"connectorIds\":[],\"side\":\"RIGHT\"},\"type\":\"ConnectorPlacement.EquallySpacedRectSide\",\"uuid\":\"385f1e4f-1c89-4afc-9c19-76a078cf90bc\"},{\"content\":{\"connectorIds\":[],\"side\":\"TOP\"},\"type\":\"ConnectorPlacement.EquallySpacedRectSide\",\"uuid\":\"fc91fa49-46f5-4ba7-960e-7bda5e0416d1\"}]},\"type\":\"ConnectorPlacement.EquallySpacedConnector\",\"uuid\":\"4bf08bc6-c7ce-47fb-af04-cd9d2b5f8092\"}],\"packageUris\":[\"http://schema.mathworks.com/mf0/Connector/19700101\"],\"version\":\"1.0\"}"
  "10.2.2.2.57\tBarrel cam position sensor wire \"GND\" insulation" : Subsystem
      settings: PortSchema="{\"entries\":[{\"content\":{\"headerSize\":26,\"margin\":15,\"minimumSpacing\":25,\"sides\":[{\"content\":{\"connectorIds\":[]},\"type\":\"ConnectorPlacement.EquallySpacedRectSide\",\"uuid\":\"f8ee33a9-954f-44c6-a821-b5353f3278fa\"},{\"content\":{\"connectorIds\":[],\"side\":\"RIGHT\"},\"type\":\"ConnectorPlacement.EquallySpacedRectSide\",\"uuid\":\"385f1e4f-1c89-4afc-9c19-76a078cf90bc\"},{\"content\":{\"connectorIds\":[],\"side\":\"TOP\"},\"type\":\"ConnectorPlacement.EquallySpacedRectSide\",\"uuid\":\"fc91fa49-46f5-4ba7-960e-7bda5e0416d1\"}]},\"type\":\"ConnectorPlacement.EquallySpacedConnector\",\"uuid\":\"4bf08bc6-c7ce-47fb-af04-cd9d2b5f8092\"}],\"packageUris\":[\"http://schema.mathworks.com/mf0/Connector/19700101\"],\"version\":\"1.0\"}"
  "10.2.2.2.58\tBarrel cam position sensor wire \"Analog Output 1\" insulation" : Subsystem
      settings: PortSchema="{\"entries\":[{\"content\":{\"headerSize\":26,\"margin\":15,\"minimumSpacing\":25,\"sides\":[{\"content\":{\"connectorIds\":[]},\"type\":\"ConnectorPlacement.EquallySpacedRectSide\",\"uuid\":\"f8ee33a9-954f-44c6-a821-b5353f3278fa\"},{\"content\":{\"connectorIds\":[],\"side\":\"RIGHT\"},\"type\":\"ConnectorPlacement.EquallySpacedRectSide\",\"uuid\":\"385f1e4f-1c89-4afc-9c19-76a078cf90bc\"},{\"content\":{\"connectorIds\":[],\"side\":\"TOP\"},\"type\":\"ConnectorPlacement.EquallySpacedRectSide\",\"uuid\":\"fc91fa49-46f5-4ba7-960e-7bda5e0416d1\"}]},\"type\":\"ConnectorPlacement.EquallySpacedConnector\",\"uuid\":\"4bf08bc6-c7ce-47fb-af04-cd9d2b5f8092\"}],\"packageUris\":[\"http://schema.mathworks.com/mf0/Connector/19700101\"],\"version\":\"1.0\"}"
  "10.2.2.2.59\tBarrel cam position sensor wire \"Analog Output 2\" insulation" : Subsystem
      settings: PortSchema="{\"entries\":[{\"content\":{\"headerSize\":26,\"margin\":15,\"minimumSpacing\":25,\"sides\":[{\"content\":{\"connectorIds\":[]},\"type\":\"ConnectorPlacement.EquallySpacedRectSide\",\"uuid\":\"f8ee33a9-954f-44c6-a821-b5353f3278fa\"},{\"content\":{\"connectorIds\":[],\"side\":\"RIGHT\"},\"type\":\"ConnectorPlacement.EquallySpacedRectSide\",\"uuid\":\"385f1e4f-1c89-4afc-9c19-76a078cf90bc\"},{\"content\":{\"connectorIds\":[],\"side\":\"TOP\"},\"type\":\"ConnectorPlacement.EquallySpacedRectSide\",\"uuid\":\"fc91fa49-46f5-4ba7-960e-7bda5e0416d1\"}]},\"type\":\"ConnectorPlacement.EquallySpacedConnector\",\"uuid\":\"4bf08bc6-c7ce-47fb-af04-cd9d2b5f8092\"}],\"packageUris\":[\"http://schema.mathworks.com/mf0/Connector/19700101\"],\"version\":\"1.0\"}"
  10.2.2.2.60	Barrel cam position sensor wires shielding braid : Subsystem
      settings: PortSchema="{\"entries\":[{\"content\":{\"headerSize\":26,\"margin\":15,\"minimumSpacing\":25,\"sides\":[{\"content\":{\"connectorIds\":[]},\"type\":\"ConnectorPlacement.EquallySpacedRectSide\",\"uuid\":\"f8ee33a9-954f-44c6-a821-b5353f3278fa\"},{\"content\":{\"connectorIds\":[],\"side\":\"RIGHT\"},\"type\":\"ConnectorPlacement.EquallySpacedRectSide\",\"uuid\":\"385f1e4f-1c89-4afc-9c19-76a078cf90bc\"},{\"content\":{\"connectorIds\":[],\"side\":\"TOP\"},\"type\":\"ConnectorPlacement.EquallySpacedRectSide\",\"uuid\":\"fc91fa49-46f5-4ba7-960e-7bda5e0416d1\"}]},\"type\":\"ConnectorPlacement.EquallySpacedConnector\",\"uuid\":\"4bf08bc6-c7ce-47fb-af04-cd9d2b5f8092\"}],\"packageUris\":[\"http://schema.mathworks.com/mf0/Connector/19700101\"],\"version\":\"1.0\"}"

== system p4_system_arch_master/System 10 : Electrical Distribution System /10.2 LV Distribution System /10.2.2	External LV Loom System/10.2.2.2	External LV loom wiring system/O Module Wires  ==

== system p4_system_arch_master/System 10 : Electrical Distribution System /10.2 LV Distribution System /10.2.2	External LV Loom System/10.2.2.3	External LV loom restraining system/10.2.2.3.1	Cable clips ==

== system p4_system_arch_master/System 2 : Gearbox System/2.1 Torque Multiplication System/2.1.5 Bearings System/Countershaft Bearings/2.1.6.0.3 B3 (NDE Countershaft Bearing)  ==

== system p4_system_arch_master/System 2 : Gearbox System/2.1 Torque Multiplication System/2.1.5 Bearings System/Countershaft Bearings/2.1.6.0.4 B4 (DE Countershaft Bearing)  ==

== system p4_system_arch_master/System 2 : Gearbox System/2.1 Torque Multiplication System/2.1.5 Bearings System/Diff Bearings/2.1.6.0.1 B1 (NDE DIff Bearing)   ==

== system p4_system_arch_master/System 2 : Gearbox System/2.1 Torque Multiplication System/2.1.5 Bearings System/Diff Bearings/2.1.6.0.2 B2 (DE DIff Bearing) ==

== system p4_system_arch_master/System 2 : Gearbox System/2.1 Torque Multiplication System/2.1.5 Bearings System/Halfshaft Bearings/2.1.6.0.10 B7 (NDE Halfshaft Bearing)  ==

== system p4_system_arch_master/System 2 : Gearbox System/2.1 Torque Multiplication System/2.1.5 Bearings System/Halfshaft Bearings/2.1.6.0.11 B8 (DE Halfshaft Bearing)  ==

== system p4_system_arch_master/System 2 : Gearbox System/2.1 Torque Multiplication System/2.1.5 Bearings System/Input Shaft Bearings/2.1.6.0.5 B5 (NDE Input Shaft Bearing)  ==

== system p4_system_arch_master/System 2 : Gearbox System/2.1 Torque Multiplication System/2.1.5 Bearings System/Input Shaft Bearings/2.1.6.0.6 B6 (DE Input Shaft Bearing) ==

== system p4_system_arch_master/System 2 : Gearbox System/2.2 Gear Shifting System/Force Transfer System 2.2.2/Fork Fixing System 2.2.2.3 /Bush 1 Fork 1 2.2.2.3.2  ==

== system p4_system_arch_master/System 2 : Gearbox System/2.2 Gear Shifting System/Force Transfer System 2.2.2/Fork Fixing System 2.2.2.3 /Bush 1 Fork 2 2.2.2.3.4  ==

== system p4_system_arch_master/System 2 : Gearbox System/2.2 Gear Shifting System/Force Transfer System 2.2.2/Fork Fixing System 2.2.2.3 /Bush 2 Fork 1 2.2.2.3.3  ==

== system p4_system_arch_master/System 2 : Gearbox System/2.2 Gear Shifting System/Force Transfer System 2.2.2/Fork Fixing System 2.2.2.3 /Bush 2 Fork 2 2.2.2.3.5  ==

== system p4_system_arch_master/System 2 : Gearbox System/2.2 Gear Shifting System/Force Transfer System 2.2.2/Fork Fixing System 2.2.2.3 /Ground Shaft 2.2.2.3.1  ==

== system p4_system_arch_master/System 2 : Gearbox System/2.2 Gear Shifting System/Force Transfer System 2.2.2/Gear Shift 1 System 2.2.2.1 /Sleeve 1 2.2.2.1.1  ==

== system p4_system_arch_master/System 2 : Gearbox System/2.2 Gear Shifting System/Force Transfer System 2.2.2/Gear Shift 2 System 2.2.2.2 /Sleeve 2 2.2.2.2.1  ==

== system p4_system_arch_master/System 2 : Gearbox System/2.2 Gear Shifting System/Torque Transfer System 2.2.1 /Actuator Gearbox 2.2.1.1 /Gear  2.2.1.1.2  ==

== system p4_system_arch_master/System 2 : Gearbox System/2.2 Gear Shifting System/Torque Transfer System 2.2.1 /Actuator Gearbox 2.2.1.1 /Gear Circlip 2.2.1.1.4  ==

== system p4_system_arch_master/System 2 : Gearbox System/2.2 Gear Shifting System/Torque Transfer System 2.2.1 /Actuator Gearbox 2.2.1.1 /Pinion 2.2.1.1.1  ==

== system p4_system_arch_master/System 2 : Gearbox System/2.2 Gear Shifting System/Torque Transfer System 2.2.1 /Actuator Gearbox 2.2.1.1 /Pinion Grub Screw 2.2.1.1.3  ==

== system p4_system_arch_master/System 2 : Gearbox System/2.2 Gear Shifting System/Torque Transfer System 2.2.1 /Drum Fixing System 2.2.1.3 /Detent Ball 2.2.1.3.3  ==

== system p4_system_arch_master/System 2 : Gearbox System/2.2 Gear Shifting System/Torque Transfer System 2.2.1 /Drum Fixing System 2.2.1.3 /Detent Body 2.2.1.3.1  ==

== system p4_system_arch_master/System 2 : Gearbox System/2.2 Gear Shifting System/Torque Transfer System 2.2.1 /Drum Fixing System 2.2.1.3 /Detent Spring 2.2.1.3.2  ==

== system p4_system_arch_master/System 2 : Gearbox System/2.2 Gear Shifting System/Torque Transfer System 2.2.1 /Torque to Force Translation 2.2.1.2 /Drum  2.2.1.2.1  ==

== system p4_system_arch_master/System 2 : Gearbox System/2.2 Gear Shifting System/Torque Transfer System 2.2.1 /Torque to Force Translation 2.2.1.2 /Drum Shims 2.2.1.2.4  ==

== system p4_system_arch_master/System 5 : Enclosure and Sealing System X/5.2 Sealing System/5.2.2 Static Seals System/5.2.2.1 Static - Flat Surface Sealing System/5.2.2.1.1 Gearbox Mating Faces Sealant ==

== system p4_system_arch_master/System 5 : Enclosure and Sealing System X/5.2 Sealing System/5.2.2 Static Seals System/5.2.2.1 Static - Flat Surface Sealing System/5.2.2.1.2 Gasket between RH Casing - Motor Cover ==

== system p4_system_arch_master/System 5 : Enclosure and Sealing System X/5.2 Sealing System/5.2.2 Static Seals System/5.2.2.1 Static - Flat Surface Sealing System/5.2.2.1.3 Gasket Between Motor Cover - Resolver Cover ==

== system p4_system_arch_master/System 5 : Enclosure and Sealing System X/5.2 Sealing System/5.2.2 Static Seals System/5.2.2.1 Static - Flat Surface Sealing System/5.2.2.1.4 Shifting Actuator Seal ==

== system p4_system_arch_master/System 5 : Enclosure and Sealing System X/5.2 Sealing System/5.2.2 Static Seals System/5.2.2.1 Static - Flat Surface Sealing System/5.2.2.1.5 LV connector Gasket ==

== system p4_system_arch_master/System 5 : Enclosure and Sealing System X/5.2 Sealing System/5.2.2 Static Seals System/5.2.2.2 Static O-Rings & Washers/5.2.2.2.1 Breather Washer ==

== system p4_system_arch_master/System 5 : Enclosure and Sealing System X/5.2 Sealing System/5.2.2 Static Seals System/5.2.2.2 Static O-Rings & Washers/5.2.2.2.10 O-ring inboard NDE cooling manifold ==

== system p4_system_arch_master/System 5 : Enclosure and Sealing System X/5.2 Sealing System/5.2.2 Static Seals System/5.2.2.2 Static O-Rings & Washers/5.2.2.2.11 O-ring between RH casing - top inverter cover ==

== system p4_system_arch_master/System 5 : Enclosure and Sealing System X/5.2 Sealing System/5.2.2 Static Seals System/5.2.2.2 Static O-Rings & Washers/5.2.2.2.12 O-Ring RH Casing - Inverter Cooling Plate ==

== system p4_system_arch_master/System 5 : Enclosure and Sealing System X/5.2 Sealing System/5.2.2 Static Seals System/5.2.2.2 Static O-Rings & Washers/5.2.2.2.13 Temperature Sensor Washer ==

== system p4_system_arch_master/System 5 : Enclosure and Sealing System X/5.2 Sealing System/5.2.2 Static Seals System/5.2.2.2 Static O-Rings & Washers/5.2.2.2.14  O-ring DC Cable Connector ==

== system p4_system_arch_master/System 5 : Enclosure and Sealing System X/5.2 Sealing System/5.2.2 Static Seals System/5.2.2.2 Static O-Rings & Washers/5.2.2.2.2 Speed Sensor LH Seal ==

== system p4_system_arch_master/System 5 : Enclosure and Sealing System X/5.2 Sealing System/5.2.2 Static Seals System/5.2.2.2 Static O-Rings & Washers/5.2.2.2.3 Oil Fill Plug Washer ==

== system p4_system_arch_master/System 5 : Enclosure and Sealing System X/5.2 Sealing System/5.2.2 Static Seals System/5.2.2.2 Static O-Rings & Washers/5.2.2.2.4 Oil drain plug washer ==

== system p4_system_arch_master/System 5 : Enclosure and Sealing System X/5.2 Sealing System/5.2.2 Static Seals System/5.2.2.2 Static O-Rings & Washers/5.2.2.2.5 RH Speed sensor seal ==

== system p4_system_arch_master/System 5 : Enclosure and Sealing System X/5.2 Sealing System/5.2.2 Static Seals System/5.2.2.2 Static O-Rings & Washers/5.2.2.2.6 O-ring Tachograph sensor ==

== system p4_system_arch_master/System 5 : Enclosure and Sealing System X/5.2 Sealing System/5.2.2 Static Seals System/5.2.2.2 Static O-Rings & Washers/5.2.2.2.7 O-ring outboard DE cooling manifold ==

== system p4_system_arch_master/System 5 : Enclosure and Sealing System X/5.2 Sealing System/5.2.2 Static Seals System/5.2.2.2 Static O-Rings & Washers/5.2.2.2.8 O-ring inboard DE cooling manifold ==

== system p4_system_arch_master/System 5 : Enclosure and Sealing System X/5.2 Sealing System/5.2.2 Static Seals System/5.2.2.2 Static O-Rings & Washers/5.2.2.2.9 O-ring outboard NDE cooling manifold ==

== system p4_system_arch_master/System 5 : Enclosure and Sealing System X/5.3 Component Enclosure Peripherals X/5.3.1 Fixing, Indexation and Labeling System/5.3.1.1 Gearbox Enclosures Fixing System/5.3.1.1.18 Capacitor fixing screws ==
  Capacitor fixing screw 1 : ModelReference  ModelNameDialog=M6x18  SimulationMode=Normal  ModelReferenceVersion=1.2
      settings: PortSchema="{\"entries\":[{\"content\":{\"headerSize\":38,\"margin\":15,\"minimumSpacing\":25,\"sides\":[{\"content\":{\"connectorIds\":[]},\"type\":\"ConnectorPlacement.EquallySpacedRectSide\",\"uuid\":\"a1de0a4a-4383-4256-97c8-b4b7017d79c3\"},{\"content\":{\"connectorIds\":[],\"side\":\"RIGHT\"},\"type\":\"ConnectorPlacement.EquallySpacedRectSide\",\"uuid\":\"b959f0e1-b665-4773-a9ab-23b80a79bba3\"},{\"content\":{\"connectorIds\":[],\"side\":\"TOP\"},\"type\":\"ConnectorPlacement.EquallySpacedRectSide\",\"uuid\":\"884e98bd-fa8a-4556-86a7-182eb6de8f96\"}]},\"type\":\"ConnectorPlacement.EquallySpacedConnector\",\"uuid\":\"31d5ce3f-6fbe-45a5-a872-1e90bd0aea01\"}],\"packageUris\":[\"http://schema.mathworks.com/mf0/Connector/19700101\"],\"version\":\"1.0\"}"
  Capacitor fixing screw 2 : ModelReference  ModelNameDialog=M6x18  SimulationMode=Normal  ModelReferenceVersion=1.2
      settings: PortSchema="{\"entries\":[{\"content\":{\"headerSize\":38,\"margin\":15,\"minimumSpacing\":25,\"sides\":[{\"content\":{\"connectorIds\":[]},\"type\":\"ConnectorPlacement.EquallySpacedRectSide\",\"uuid\":\"a1de0a4a-4383-4256-97c8-b4b7017d79c3\"},{\"content\":{\"connectorIds\":[],\"side\":\"RIGHT\"},\"type\":\"ConnectorPlacement.EquallySpacedRectSide\",\"uuid\":\"b959f0e1-b665-4773-a9ab-23b80a79bba3\"},{\"content\":{\"connectorIds\":[],\"side\":\"TOP\"},\"type\":\"ConnectorPlacement.EquallySpacedRectSide\",\"uuid\":\"884e98bd-fa8a-4556-86a7-182eb6de8f96\"}]},\"type\":\"ConnectorPlacement.EquallySpacedConnector\",\"uuid\":\"31d5ce3f-6fbe-45a5-a872-1e90bd0aea01\"}],\"packageUris\":[\"http://schema.mathworks.com/mf0/Connector/19700101\"],\"version\":\"1.0\"}"
